simulink model "test_"  (R2015a)
settings: Solver=ode3  StartTime=0.0  StopTime=inf  RelTol=1e-3
libraries: PoliArd x9
settings Model: ExtModeTrigDuration=2  Creator=user  LastModifiedBy=lelli
settings OptimizationCC: OptimizeModelRefInitCode=on  LifeSpan=1
settings DebuggingCC: UnderspecifiedInitializationDetection=Classic  MergeDetectMultiDrivingBlocksExec=none
settings HardwareCC: ProdLargestAtomicInteger=Long  ProdLargestAtomicFloat=Double  ProdEndianess=LittleEndian  ProdHWDeviceType=ARM Compatible->ARM Cortex
settings RTWCC: SystemTargetFile=realtime.tlc  GenerateMakefile=off  TemplateMakefile=realtime.tmf  Description=Run on Target Hardware  RTWVerbose=off
settings ERTTargetCC: CombineOutputUpdateFcns=off  ExtModeTransport=3  ExtModeMexFile=ext_serial_win32_comm_rtt  ExtModeMexArgs=0 1 9600  ERTSrcFileBannerTemplate=realtime_code_template.cgt  ERTHdrFileBannerTemplate=realtime_code_template.cgt  ERTDataSrcFileTemplate=realtime_code_template.cgt  ERTDataHdrFileTemplate=realtime_code_template.cgt  ERTCustomFileTemplate=realtime_file_process.tlc

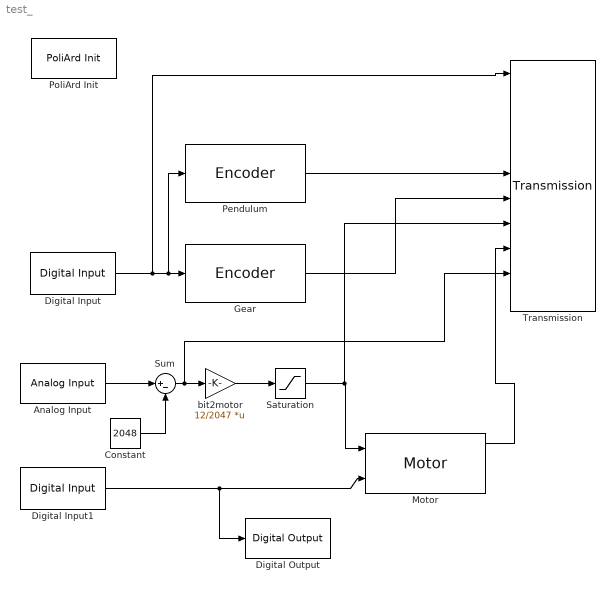
== system test_ ==
  Analog Input : PoliArd/Analog Input  AIpin_mask=8  AIsample=-1
  Constant : Constant  Value=2048
  Digital Input : PoliArd/Digital Input  DI_pin=2  DIsample=-1
  Digital Input1 : PoliArd/Digital Input  DI_pin=3  DIsample=-1
  Digital Output : PoliArd/Digital Output  DO_pin=1
  Gear : PoliArd/Encoder  EncoderID=3  dt_enc=-1
  Motor : PoliArd/Motor  MotorID=1  DC_bus_mask=12  dt_mot=-1
  "Pendulum " : PoliArd/Encoder  EncoderID=1  dt_enc=-1
  PoliArd Init : PoliArd/PoliArd Init
  Saturation : Saturate  UpperLimit=12  LowerLimit=-12
  Sum : Sum  Inputs=|+-
  Transmission : PoliArd/Transmission  sample_freq=100  sig_to_send=6
  bit2motor : Gain  Gain=12/2047  Multiplication=Matrix(K*u)
  wires:
  "Pendulum "/1 -> Transmission/5
  Gear/1 -> Transmission/6
  Digital Input1/1 -> Digital Output/1, Motor/2
  Analog Input/1 -> Sum/1
  Constant/1 -> Sum/2
  Sum/1 -> Transmission/9, bit2motor/1
  bit2motor/1 -> Saturation/1
  Motor/1 -> Transmission/8
  Saturation/1 -> Transmission/7, Motor/1
  Digital Input/1 -> Transmission/1, "Pendulum "/1, Gear/1
